simulink model "Linear_regression_ISMC_CP"  (R2021b)
settings: Solver=ode3  StartTime=0.0  StopTime=50  FixedStep=0.01  RelTol=1e-3
values from neighbouring files (symbols this model uses):
  c1 = par(pop_index,1)    [GA_Sliding.m]    (also in running_simulation_LinearRegressiomISMCCP.m = 232.921)
  c2 = par(pop_index,2)    [GA_Sliding.m]    (also in running_simulation_LinearRegressiomISMCCP.m = 254.559)
  c3 = par(pop_index,3)    [GA_Sliding.m]    (also in running_simulation_LinearRegressiomISMCCP.m = -910.366)
  c4 = par(pop_index,4)    [GA_Sliding.m]    (also in running_simulation_LinearRegressiomISMCCP.m = -279.992)
  k = par(pop_index,5)    [GA_Sliding.m]    (also in running_simulation_LinearRegressiomISMCCP.m = 150)
  period = 20    [running_simulation_LinearRegressiomISMCCP.m]
  x1_init = 0    [running_simulation_LinearRegressiomISMCCP.m]
  x2_init = 0.1    [running_simulation_LinearRegressiomISMCCP.m]
  x3_init = 0.2    [running_simulation_LinearRegressiomISMCCP.m]
  x4_init = 0    [running_simulation_LinearRegressiomISMCCP.m]
  x_1 = 30    [running_simulation_LinearRegressiomISMCCP.m]
  x_10 = 0    [running_simulation_LinearRegressiomISMCCP.m]
  x_2 = 15    [running_simulation_LinearRegressiomISMCCP.m]
  x_3 = 8    [running_simulation_LinearRegressiomISMCCP.m]
  x_4 = 7    [running_simulation_LinearRegressiomISMCCP.m]
  x_5 = 6    [running_simulation_LinearRegressiomISMCCP.m]
  x_6 = 5    [running_simulation_LinearRegressiomISMCCP.m]
  x_7 = 4    [running_simulation_LinearRegressiomISMCCP.m]
  x_8 = 3    [running_simulation_LinearRegressiomISMCCP.m]
  x_9 = 2    [running_simulation_LinearRegressiomISMCCP.m]
settings Model: Creator=ASUS  LastModifiedBy=bao04
settings SolverCC: AlgebraicLoopSolver=TrustRegion
settings DataIOCC: ReturnWorkspaceOutputs=off
settings DebuggingCC: SFMachineParentedDataDiag=warning  ArithmeticOperatorsInVariantConditions=warning
settings SFSimCC: SimUseLocalCustomCode=off  CustomCodeUndefinedFunction=UseInterfaceOnly
settings RTWCC: RTWUseLocalCustomCode=off
settings CodeAppCC: StateflowObjectComments=on

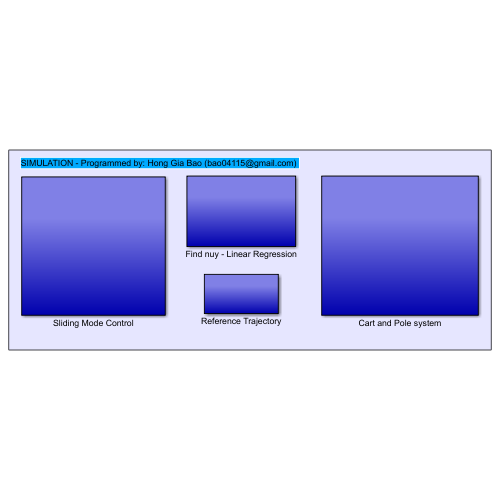
[thumbnail: Simulink's stored preview of the top-level diagram]
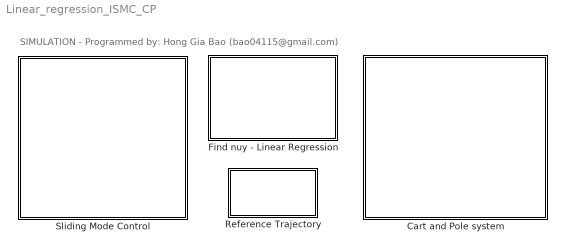
== system Linear_regression_ISMC_CP ==
  note: SIMULATION - Programmed by: Hong Gia Bao (bao04115@gmail.com)
  Cart and Pole system : Subsystem
  Find nuy - Linear Regression : Subsystem
  Reference Trajectory : Subsystem
  Sliding Mode Control : Subsystem

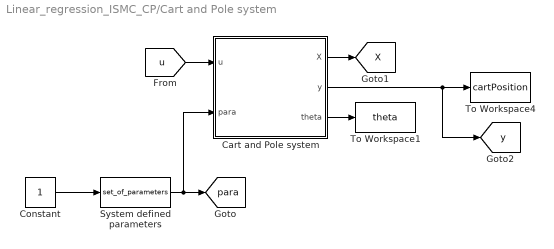
== system Linear_regression_ISMC_CP/Cart and Pole system ==
  Cart and Pole system : Subsystem
  Constant : Constant
  System defined parameters : MATLABFcn  MATLABFcn=set_of_parameters
  To Workspace1 : ToWorkspace  VariableName=theta  SaveFormat=Timeseries  SampleTime=-1
  To Workspace4 : ToWorkspace  VariableName=cartPosition  SaveFormat=Timeseries  SampleTime=-1
  tag scope: X=global, para=global, y=global
  wires:
  [u] -> Cart and Pole system/1(u)
  Cart and Pole system/1(X) -> [X]
  Cart and Pole system/3(theta) -> To Workspace1/1
  Cart and Pole system/2(y) -> [y], To Workspace4/1
  Constant/1 -> System defined parameters/1
  System defined parameters/1 -> Cart and Pole system/2(para), [para]

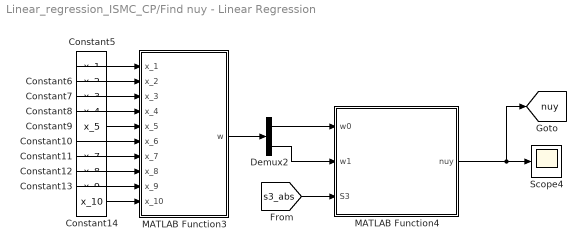
== system Linear_regression_ISMC_CP/Find nuy - Linear Regression ==
  Constant10 : Constant  Value=x_6
  Constant11 : Constant  Value=x_7
  Constant12 : Constant  Value=x_8
  Constant13 : Constant  Value=x_9
  Constant14 : Constant  Value=x_10
  Constant5 : Constant  Value=x_1
  Constant6 : Constant  Value=x_2
  Constant7 : Constant  Value=x_3
  Constant8 : Constant  Value=x_4
  Constant9 : Constant  Value=x_5
  Demux2 : Demux  Outputs=2
  MATLAB Function3 : MATLAB Function  TreatAsAtomicUnit=on
  MATLAB Function4 : MATLAB Function  TreatAsAtomicUnit=on
  Scope4 : Scope
  tag scope: nuy=global
  wires:
  Constant8/1 -> MATLAB Function3/4(x_4)
  Constant6/1 -> MATLAB Function3/2(x_2)
  Constant10/1 -> MATLAB Function3/6(x_6)
  Constant5/1 -> MATLAB Function3/1(x_1)
  Constant7/1 -> MATLAB Function3/3(x_3)
  Constant9/1 -> MATLAB Function3/5(x_5)
  Constant12/1 -> MATLAB Function3/8(x_8)
  MATLAB Function4/1(nuy) -> [nuy], Scope4/1
  Constant11/1 -> MATLAB Function3/7(x_7)
  MATLAB Function3/1(w) -> Demux2/1
  Constant13/1 -> MATLAB Function3/9(x_9)
  Demux2/2 -> MATLAB Function4/2(w1)
  Demux2/1 -> MATLAB Function4/1(w0)
  Constant14/1 -> MATLAB Function3/10(x_10)
  [s3_abs] -> MATLAB Function4/3(S3)

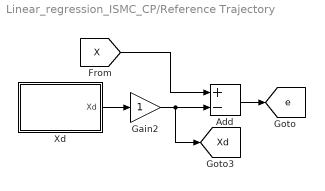
== system Linear_regression_ISMC_CP/Reference Trajectory ==
  Add : Sum  Inputs=+-
  Gain2 : Gain
  Xd : Subsystem
  tag scope: Xd=global, e=global
  wires:
  [X] -> Add/1
  Add/1 -> [e]
  Xd/1(Xd) -> Gain2/1
  Gain2/1 -> [Xd], Add/2

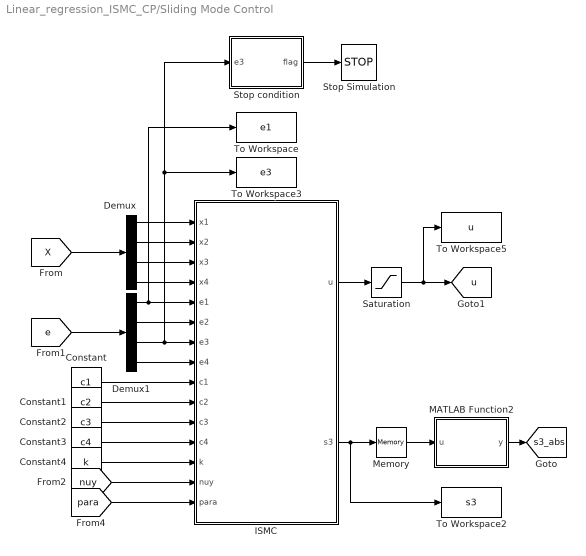
== system Linear_regression_ISMC_CP/Sliding Mode Control ==
  Constant : Constant  Value=c1
  Constant1 : Constant  Value=c2
  Constant2 : Constant  Value=c3
  Constant3 : Constant  Value=c4
  Constant4 : Constant  Value=k
  Demux : Demux
  Demux1 : Demux
  ISMC : MATLAB Function  TreatAsAtomicUnit=on
  MATLAB Function2 : MATLAB Function  TreatAsAtomicUnit=on
  Memory : Memory
  Saturation : Saturate  UpperLimit=24  LowerLimit=-24
  Stop Simulation : Stop
  Stop condition : MATLAB Function  TreatAsAtomicUnit=on
  To Workspace : ToWorkspace  VariableName=e1  SampleTime=-1
  To Workspace2 : ToWorkspace  VariableName=s3  SampleTime=-1
  To Workspace3 : ToWorkspace  VariableName=e3  SampleTime=-1
  To Workspace5 : ToWorkspace  VariableName=u  SampleTime=-1
  tag scope: s3_abs=global, u=global
  wires:
  Saturation/1 -> To Workspace5/1, [u]
  Demux/2 -> ISMC/2(x2)
  Demux/1 -> ISMC/1(x1)
  Constant/1 -> ISMC/9(c1)
  [X] -> Demux/1
  Demux1/1 -> To Workspace/1, ISMC/5(e1)
  ISMC/1(u) -> Saturation/1
  Demux1/2 -> ISMC/6(e2)
  [e] -> Demux1/1
  Demux/3 -> ISMC/3(x3)
  Demux1/4 -> ISMC/8(e4)
  Stop condition/1(flag) -> Stop Simulation/1
  Constant2/1 -> ISMC/11(c3)
  Constant1/1 -> ISMC/10(c2)
  Demux/4 -> ISMC/4(x4)
  Constant3/1 -> ISMC/12(c4)
  Demux1/3 -> Stop condition/1(e3), To Workspace3/1, ISMC/7(e3)
  Constant4/1 -> ISMC/13(k)
  ISMC/2(s3) -> To Workspace2/1, Memory/1
  MATLAB Function2/1(y) -> [s3_abs]
  Memory/1 -> MATLAB Function2/1(u)
  [nuy] -> ISMC/14(nuy)
  [para] -> ISMC/15(para)

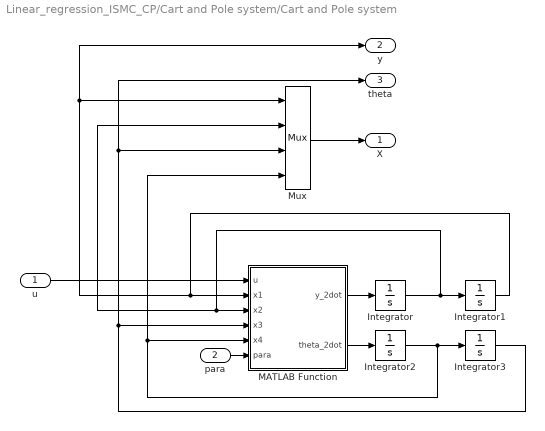
== system Linear_regression_ISMC_CP/Cart and Pole system/Cart and Pole system ==
  u : Inport
  para : Inport  Port=2
  Integrator : Integrator  InitialCondition=x2_init
  Integrator1 : Integrator  InitialCondition=x1_init
  Integrator2 : Integrator  InitialCondition=x4_init
  Integrator3 : Integrator  InitialCondition=x3_init
  MATLAB Function : MATLAB Function  TreatAsAtomicUnit=on
  Mux : Mux
  X : Outport
  y : Outport  Port=2
  theta : Outport  Port=3
  wires:
  u/1 -> MATLAB Function/1(u)
  Integrator/1 -> MATLAB Function/3(x2), Mux/2, Integrator1/1
  Integrator2/1 -> Integrator3/1, Mux/4, MATLAB Function/5(x4)
  MATLAB Function/2(theta_2dot) -> Integrator2/1
  MATLAB Function/1(y_2dot) -> Integrator/1
  Mux/1 -> X/1
  Integrator1/1 -> MATLAB Function/2(x1), Mux/1, y/1
  Integrator3/1 -> MATLAB Function/4(x3), theta/1, Mux/3
  para/1 -> MATLAB Function/6(para)

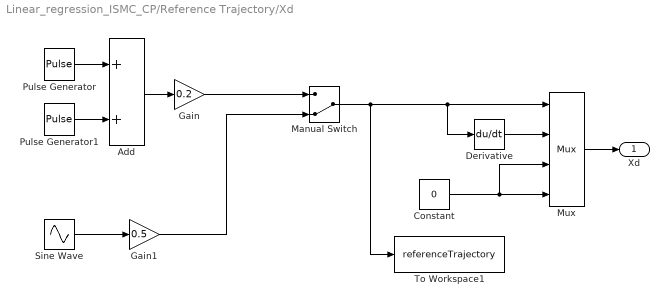
== system Linear_regression_ISMC_CP/Reference Trajectory/Xd ==
  Add : Sum
  Constant : Constant  Value=0
  Derivative : Derivative
  Gain : Gain  Gain=0.2
  Gain1 : Gain  Gain=0.5
  Manual Switch : ManualSwitch  CurrentSetting=0
  Mux : Mux
  Pulse Generator : DiscretePulseGenerator  PulseType=Time based  Period=period  PulseWidth=50
  Pulse Generator1 : DiscretePulseGenerator  PulseType=Time based  Amplitude=-1  Period=period  PulseWidth=50  PhaseDelay=period/2
  Sine Wave : Sin  Frequency=2*pi/period
  To Workspace1 : ToWorkspace  VariableName=referenceTrajectory  SaveFormat=Timeseries  SampleTime=-1
  Xd : Outport
  wires:
  Pulse Generator/1 -> Add/1
  Add/1 -> Gain/1
  Pulse Generator1/1 -> Add/2
  Mux/1 -> Xd/1
  Constant/1 -> Mux/4, Mux/3
  Manual Switch/1 -> To Workspace1/1, Derivative/1, Mux/1
  Gain/1 -> Manual Switch/1
  Sine Wave/1 -> Gain1/1
  Derivative/1 -> Mux/2
  Gain1/1 -> Manual Switch/2

== matlab function Linear_regression_ISMC_CP/Sliding Mode Control/ISMC ==
  data: x1 input; u output; x2 input; x3 input; x4 input; e1 input; e2 input; e3 input; e4 input; c1 input; c2 input; c3 input; c4 input; k input; s3 output; nuy input; para input
function [u,s3] = fcn(x1,x2,x3,x4,e1,e2,e3,e4,c1,c2,c3,c4,k,nuy, para)

mc      = para(1);
m       = para(2);
l       = para(3);  
a       = para(4);
g       = para(5);
I       = para(6);
Kb      = para(7);
Rm      = para(9);
Jm      = para(10);
Cm      = para(11);
Radius  = para(12);
k1      = para(13);
k2      = para(14);
k3      = para(15);

f1      = (- sin(x3)*a^3*m^2*x4^2 + g*cos(x3)*sin(x3)*a^2*m^2 + k2*x2*a^2*m - I*sin(x3)*a*m*x4^2 + I*k2*x2)/(I*m - I*k3 + I*mc + a^2*m^2 - a^2*m^2*cos(x3)^2 - a^2*k3*m + a^2*m*mc);
f2      = (a*m*(- a*m*cos(x3)*sin(x3)*x4^2 - g*k3*sin(x3) + k2*x2*cos(x3) + g*m*sin(x3) + g*mc*sin(x3)))/(I*m - I*k3 + I*mc + a^2*m^2 - a^2*m^2*cos(x3)^2 - a^2*k3*m + a^2*m*mc);
b1      = (k1*(m*a^2 + I))/(I*m - I*k3 + I*mc + a^2*m^2*sin(x3)^2 - a^2*k3*m + a^2*m*mc);
b2      = (a*k1*m*cos(x3))/(I*m - I*k3 + I*mc + a^2*m^2 - a^2*m^2*cos(x3)^2 - a^2*k3*m + a^2*m*mc);

% sliding surfaces  
s1      = c1*e1 + c2*e2;
s2      = s1 + c3*e3;
s3      = s2 + c4*e4;

% control input
u       = (-1)/(c4*b2+c2*b1)*(c4*f2-(-c3)*x4-(-c1)*x2+c2*f1+(nuy*sign(s3)+k*s3));

== matlab function Linear_regression_ISMC_CP/Cart and Pole system/Cart and Pole system/MATLAB Function ==
  data: u input; y_2dot output; x1 input; x2 input; x3 input; x4 input; theta_2dot output; para input
function [y_2dot, theta_2dot]= fcn(u,x1,x2,x3,x4,para)

mc      = para(1);
m       = para(2);
l       = para(3);  
a       = para(4);
g       = para(5);
I       = para(6);
Kb      = para(7);
Rm      = para(9);
Jm      = para(10);
Cm      = para(11);
Radius  = para(12);
k1      = para(13); 
k2      = para(14); 
k3      = para(15); 

y_2dot      = (I*x2*k2 + I*k1*u + x2*a^2*k2*m + a^2*k1*m*u - a^3*m^2*x4^2*sin(x3) + a^2*g*m^2*cos(x3)*sin(x3) ...
               - I*a*m*x4^2*sin(x3))/(I*m - I*k3 + I*mc + a^2*m^2 - a^2*m^2*cos(x3)^2 - a^2*k3*m + a^2*m*mc);
theta_2dot  = (a*m*(- a*m*cos(x3)*sin(x3)*x4^2 + k1*u*cos(x3) - g*k3*sin(x3) + g*m*sin(x3) + g*mc*sin(x3) ...
               + x2*k2*cos(x3)))/(I*m - I*k3 + I*mc + a^2*m^2 - a^2*m^2*cos(x3)^2 - a^2*k3*m + a^2*m*mc);

== matlab function Linear_regression_ISMC_CP/Sliding Mode Control/Stop condition ==
  data: flag output; e3 input
function flag = fcn(e3)
    if abs(e3) > 3
        flag = 1;
    else
        flag = 0;
    end

== matlab function Linear_regression_ISMC_CP/Sliding Mode Control/MATLAB Function2 ==
  data: u input; y output
function y = fcn(u)

y = abs(u);

== matlab function Linear_regression_ISMC_CP/Find nuy - Linear Regression/MATLAB Function3 ==
  data: w output; x_1 input; x_2 input; x_3 input; x_4 input; x_5 input; x_6 input; x_7 input; x_8 input; x_9 input; x_10 input
function w  = fcn(x_1,x_2,x_3,x_4,x_5,x_6,x_7,x_8,x_9,x_10)

X1  = [x_1,x_2,x_3,x_4,x_5,x_6,x_7,x_8,x_9,x_10]';
X0  = ones(size(X1),'like',X1);
y   = [9,8,7,6,5,4,3,2,1,0];

Xbar    = [X0,X1];
A       = Xbar'*Xbar;
B       = Xbar'*y';
w       = pinv(A)*B;

== matlab function Linear_regression_ISMC_CP/Find nuy - Linear Regression/MATLAB Function4 ==
  data: w0 input; nuy output; w1 input; S3 input
function nuy = fcn(w0,w1,S3)
   
    if S3<18
        nuy = w0+w1*S3;
    else if S3 ==0
        nuy = 0;
        else 
            nuy =20;
        end
    end
